simulink model "MerArbiter"  (Simulink 7.1)
settings: Solver=ode45  StartTime=0.0  StopTime=inf  RelTol=1e-3
settings Model: Creator=daniel  LastModifiedBy=cpasarea
settings DebuggingCC: SaveWithParameterizedLinksMsg=none  SignalResolutionControl=TryResolveAllWithWarning  MultiTaskDSMMsg=warning  MultiTaskCondExecSysMsg=none
settings RTWCC: IncludeERTFirstTime=on
settings GRTTargetCC: TargetFcnLib=ansi_tfl_tmw.mat

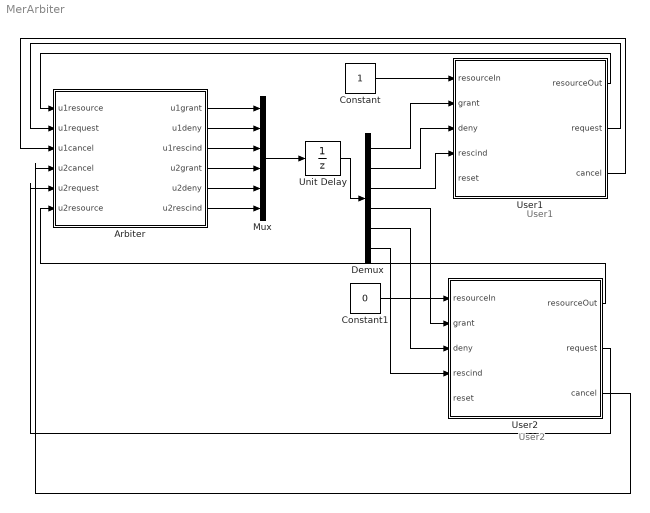
== system MerArbiter ==
  note: User2
  note: User1
  Arbiter : Stateflow chart  TreatAsAtomicUnit=on
  Constant : Constant  OutDataTypeMode=uint8  OutDataTypeStr=uint8
  Constant1 : Constant  Value=0  OutDataTypeMode=uint8  OutDataTypeStr=uint8
  Demux : Demux  Outputs=6
  Mux : Mux  Inputs=6
  Unit Delay : UnitDelay  X0=[false,false,false,false,false,false]  SampleTime=-1
  User1 : Stateflow chart  TreatAsAtomicUnit=on
  User2 : Stateflow chart  TreatAsAtomicUnit=on
  wires:
  Arbiter/1(u1grant) -> Mux/1
  Arbiter/2(u1deny) -> Mux/2
  Arbiter/3(u1rescind) -> Mux/3
  Arbiter/4(u2grant) -> Mux/4
  Arbiter/5(u2deny) -> Mux/5
  Arbiter/6(u2rescind) -> Mux/6
  Mux/1 -> Unit Delay/1
  Unit Delay/1 -> Demux/1
  Constant1/1 -> User2/1(resourceIn)
  Demux/4 -> User2/2(grant)
  Demux/5 -> User2/3(deny)
  Demux/6 -> User2/4(rescind)
  User2/1(resourceOut) -> Arbiter/6(u2resource)
  User2/2(request) -> Arbiter/5(u2request)
  User2/3(cancel) -> Arbiter/4(u2cancel)
  Constant/1 -> User1/1(resourceIn)
  Demux/1 -> User1/2(grant)
  Demux/2 -> User1/3(deny)
  Demux/3 -> User1/4(rescind)
  User1/1(resourceOut) -> Arbiter/1(u1resource)
  User1/2(request) -> Arbiter/2(u1request)
  User1/3(cancel) -> Arbiter/3(u1cancel)

== stateflow chart Arbiter ==
  settings: updateMethod=DISCRETE  sampleTime=1
  state Init
  state Running
    state User1 [parallel]
      settings: executionOrder=2
      state Idle
      state Comm
        en: u1grant = true;
        u1deny = false;
        resources[commUser] = 1;
      state WaitForCancel
      state Drive
        en: u1grant = true;
        u1deny = false;
        resources[driveUser] = 1;
      state Arm
        en: u1grant = true;
        u1deny = false;
        resources[armUser] = 1;
      state Rat
        en: u1grant = true;
        u1deny = false;
        resources[ratUser] = 1;
      state PanCam
        en: u1grant = true;
        u1deny = false;
        resources[panCamUser] = 1;
      Running.User1.WaitForCancel -> Running.User1.Comm : [u2cancel == true]
      (junction 21) -> Running.User1.Comm [order 1] : [u1resource == commUser && ...
          | resources[commUser] == 0 && ...
          | resources[driveUser] == 0 ]
      (junction 21) -> Running.User1.Idle [order 2] : [resources[commUser] != 0] {u1deny = true; u1grant = false;}
      (junction 21) -> (junction 23) [order 3]
      Running.User1.Idle -> (junction 22) : [u1request == true]
      (junction 22) -> (junction 21) [order 1] : [u1resource == commUser]
      (junction 23) -> Running.User1.WaitForCancel : [resources[driveUser] == 2] {u2rescind = true;}
      (junction 31) -> (junction 32) [order 2]
      (junction 22) -> (junction 24) [order 2]
      (junction 24) -> (junction 25) [order 1] : [u1resource == driveUser]
      (junction 25) -> Running.User1.Drive [order 1] : [resources[commUser] == 0 && ...
          | resources[driveUser] == 0 ]
      (junction 25) -> (junction 32) [order 2]
      Running.User1.Comm -> Running.User1.Idle : [u1cancel == true] {resources[commUser] = 0;}
      (junction 24) -> (junction 26) [order 2]
      (junction 26) -> (junction 27) [order 1] : [u1resource == armUser]
      (junction 27) -> Running.User1.Arm [order 1] : [resources[armUser] == 0 && ...
          | resources[ratUser] == 0  && ...
          | resources[panCamUser] == 0 ]
      (junction 26) -> (junction 28) [order 2]
      (junction 28) -> (junction 29) [order 1] : [u1resource == ratUser]
      (junction 29) -> Running.User1.Rat [order 1] : [resources[armUser] == 0 && ...
          | resources[ratUser] == 0 && ...
          | resources[commUser] == 0]
      (junction 28) -> (junction 30) [order 2]
      (junction 30) -> (junction 31) : [u1resource == panCamUser]
      (junction 31) -> Running.User1.PanCam [order 1] : [resources[armUser] == 0 && ...
          | resources[panCamUser] == 0]
      (junction 27) -> (junction 32) [order 2]
      (junction 29) -> (junction 32) [order 2]
      Running.User1.Drive -> (junction 33) : [u1cancel == true] {resources[driveUser] = 0;}
      Running.User1.Arm -> (junction 34) : [u1cancel == true] {resources[armUser] = 0;}
      Running.User1.Rat -> (junction 35) : [u1cancel == true] {resources[ratUser] = 0;}
      Running.User1.PanCam -> (junction 36) : [u1cancel == true] {resources[panCamUser] = 0;}
      (junction 36) -> (junction 35)
      (junction 35) -> (junction 34)
      (junction 34) -> (junction 33)
      (junction 33) -> Running.User1.Idle
      (default) -> Running.User1.Idle
    state User2 [parallel]
      settings: executionOrder=1
      state Idle
      state Comm
        en: u2grant = true;
        u2deny = false;
        resources[commUser] = 2;
      state WaitForCancel
      state Drive
        en: u2grant = true;
        u2deny = false;
        resources[driveUser] = 2;
      state Arm
        en: u2grant = true;
        u2deny = false;
        resources[armUser] = 2;
      state Rat
        en: u2grant = true;
        u2deny = false;
        resources[ratUser] = 2;
      state PanCam
        en: u2grant = true;
        u2deny = false;
        resources[panCamUser] = 2;
      Running.User2.WaitForCancel -> Running.User2.Comm : [u2cancel == true]
      (junction 37) -> Running.User2.Comm [order 1] : [u2resource == commUser && ...
          | resources[commUser] == 0 && ...
          | resources[driveUser] == 0 ]
      (junction 37) -> Running.User2.Idle [order 2] : [resources[commUser] != 0] {u1deny = true; u1grant = false;}
      (junction 37) -> (junction 39) [order 3]
      Running.User2.Idle -> (junction 38) : [u2request == true]
      (junction 38) -> (junction 37) [order 1] : [u2resource == commUser]
      (junction 39) -> Running.User2.WaitForCancel : [resources[driveUser] == 1] {u1rescind = true;}
      (junction 38) -> (junction 40) [order 2]
      (junction 40) -> (junction 41) [order 1] : [u2resource == driveUser]
      (junction 41) -> Running.User2.Drive [order 1] : [resources[commUser] == 0 && ...
          | resources[driveUser] == 0 ]
      (junction 40) -> (junction 42) [order 2]
      (junction 42) -> (junction 43) [order 1] : [u2resource == armUser]
      (junction 43) -> Running.User2.Arm [order 1] : [resources[armUser] == 0 && ...
          | resources[ratUser] == 0&& ...
          | resources[panCamUser] == 0]
      (junction 42) -> (junction 44) [order 2]
      (junction 44) -> (junction 45) [order 1] : [u2resource == ratUser]
      (junction 45) -> Running.User2.Rat [order 1] : [resources[armUser] == 0 && ...
          | resources[ratUser] == 0 && ...
          | resources[commUser] == 0]
      (junction 44) -> (junction 49) [order 2]
      (junction 43) -> (junction 46) [order 2]
      (junction 45) -> (junction 46) [order 2]
      (junction 50) -> (junction 46) [order 2]
      (junction 41) -> (junction 46) [order 2]
      Running.User2.Comm -> Running.User2.Idle : [u2cancel == true] {resources[commUser] = 0;}
      Running.User2.Drive -> (junction 47) : [u2cancel == true] {resources[driveUser] = 0;}
      Running.User2.Arm -> (junction 48) : [u2cancel == true] {resources[armUser] = 0;}
      (junction 51) -> (junction 48)
      (junction 48) -> (junction 47)
      (junction 47) -> Running.User2.Idle
      (junction 49) -> (junction 50) : [u2resource == panCamUser]
      (junction 50) -> Running.User2.PanCam [order 1] : [resources[armUser] == 0 && ...
          | resources[panCamUser] == 0 ]
      Running.User2.Rat -> (junction 51) : [u2cancel == true] {resources[ratUser] = 0;}
      Running.User2.PanCam -> (junction 52) : [u2cancel == true] {resources[panCamUser] = 0;}
      (junction 52) -> (junction 51)
      (default) -> Running.User2.Idle
  (default) -> Init : {commUser = 0; driveUser = 1; panCamUser = 2; armUser = 3; ratUser = 4;
      | resources[commUser] = 0; resources[driveUser] = 0;
      | resources[panCamUser] = 0; resources[armUser] = 0; resources[ratUser] =0;}
  Init -> Running
  data: commUser local uint8; driveUser local uint8; panCamUser local uint8; armUser local uint8; ratUser local uint8; u1resource input uint8 size=1; u1request input boolean; u1cancel input boolean; u1grant output boolean; u1deny output boolean; u1rescind output boolean; resources local uint8 size=5; u2cancel input boolean; u2request input boolean; u2resource input uint8 size=1; u2grant output boolean; u2deny output boolean; u2rescind output boolean

== stateflow chart User1 ==
  settings: updateMethod=DISCRETE  sampleTime=1
  state Idle
  state Busy
    state Init
    state Pending
    state Granted
    Granted -> Init [order 1] : [rescind == true] {cancel = true}
    Pending -> Granted [order 2] : [grant == true]
    (default) -> Init
    Init -> Pending : {request = true}
    Pending -> Init [order 1] : [deny == true]...
        | {request = false}
  Busy -> Idle : [reset == true] ...
      | {cancel = true; request = false;}
  Idle -> Busy : [resourceIn >=0 && resourceIn < 5] ...
      | {resourceOut = resourceIn; cancel = false;}
  (default) -> Idle
  Granted -> Idle [order 2] : {cancel = true; request = false;}
  data: resourceIn input uint8; resourceOut output uint8; request output boolean; grant input boolean; cancel output boolean; deny input boolean; rescind input boolean; reset input boolean

== stateflow chart User2 ==
  settings: updateMethod=DISCRETE  sampleTime=1
  state Idle
  state Busy
    state Init
    state Pending
    state Granted
    Granted -> Init [order 1] : [rescind == true] {cancel = true}
    Pending -> Granted [order 2] : [grant == true]
    (default) -> Init
    Init -> Pending : {request = true}
    Pending -> Init [order 1] : [deny == true]...
        | {request = false}
  Busy -> Idle : [reset == true] ...
      | {cancel = true; request = false;}
  Idle -> Busy : [resourceIn >=0 && resourceIn < 5] ...
      | {resourceOut = resourceIn; cancel = false;}
  (default) -> Idle
  Granted -> Idle [order 2] : {cancel = true; request = false;}
  data: resourceIn input uint8; resourceOut output uint8; request output boolean; grant input boolean; cancel output boolean; deny input boolean; rescind input boolean; reset input boolean
